simulink library "halin"  (R2021b)
settings: Solver=VariableStepAuto  StartTime=0.0  StopTime=10.0  RelTol=1e-3
undefined symbols (not defined in the file): TRUE
libraries: FVT_lib x100, hcu_lib x41
(part 4 of 10)

== system halin/HAL_IN/CAN1/EBC5 ==
  DT_CAN1_SG_EBC5 : Inport
  BrkTempeWarn : Subsystem
  FndBrkUse : Subsystem
  HaltBrkMode : Subsystem
  HillHolderMode : Subsystem
  ParkBrkActuFAct : Subsystem
  XBRAcltnLimit : Subsystem
  XBRActtrlMode : Subsystem
  XBRSysSta : Subsystem
  bus_selector : BusSelector  OutputSignals=CAN1_BrkTempeWarn
  bus_selector1 : BusSelector  OutputSignals=CAN1_FndBrkUse
  bus_selector2 : BusSelector  OutputSignals=CAN1_HaltBrkMode
  bus_selector3 : BusSelector  OutputSignals=CAN1_HillHolderMode
  bus_selector4 : BusSelector  OutputSignals=CAN1_ParkBrkActuFAct
  bus_selector5 : BusSelector  OutputSignals=CAN1_XBRAcltnLimit
  bus_selector6 : BusSelector  OutputSignals=CAN1_XBRActtrlMode
  bus_selector7 : BusSelector  OutputSignals=CAN1_XBRSysSta
  VHAL_BrkTempeWarn_enum : Outport
  VHAL_FndBrkUse_enum : Outport  Port=2
  VHAL_HaltBrkMode_enum : Outport  Port=3
  VHAL_HillHolderMode_enum : Outport  Port=4
  VHAL_ParkBrkActuFAct_enum : Outport  Port=5
  VHAL_XBRAcltnLimit_mps2 : Outport  Port=6
  VHAL_XBRActtrlMode_enum : Outport  Port=7
  VHAL_XBRSysSta_enum : Outport  Port=8
  wires:
  DT_CAN1_SG_EBC5/1 -> [DT_CAN1_SG_EBC5]
  [DT_CAN1_SG_EBC5] -> bus_selector/1
  bus_selector/1 -> BrkTempeWarn/1(BrkTempeWarn)  "<CAN1_BrkTempeWarn>"
  BrkTempeWarn/1(VHAL_BrkTempeWarn_enum) -> VHAL_BrkTempeWarn_enum/1
  [DT_CAN1_SG_EBC5] -> bus_selector1/1
  bus_selector1/1 -> FndBrkUse/1(FndBrkUse)  "<CAN1_FndBrkUse>"
  FndBrkUse/1(VHAL_FndBrkUse_enum) -> VHAL_FndBrkUse_enum/1
  [DT_CAN1_SG_EBC5] -> bus_selector2/1
  bus_selector2/1 -> HaltBrkMode/1(HaltBrkMode)  "<CAN1_HaltBrkMode>"
  HaltBrkMode/1(VHAL_HaltBrkMode_enum) -> VHAL_HaltBrkMode_enum/1
  [DT_CAN1_SG_EBC5] -> bus_selector3/1
  bus_selector3/1 -> HillHolderMode/1(HillHolderMode)  "<CAN1_HillHolderMode>"
  HillHolderMode/1(VHAL_HillHolderMode_enum) -> VHAL_HillHolderMode_enum/1
  [DT_CAN1_SG_EBC5] -> bus_selector4/1
  bus_selector4/1 -> ParkBrkActuFAct/1(ParkBrkActuFAct)  "<CAN1_ParkBrkActuFAct>"
  ParkBrkActuFAct/1(VHAL_ParkBrkActuFAct_enum) -> VHAL_ParkBrkActuFAct_enum/1
  [DT_CAN1_SG_EBC5] -> bus_selector5/1
  bus_selector5/1 -> XBRAcltnLimit/1(XBRAcltnLimit)  "<CAN1_XBRAcltnLimit>"
  XBRAcltnLimit/1(VHAL_XBRAcltnLimit_mps2) -> VHAL_XBRAcltnLimit_mps2/1
  [DT_CAN1_SG_EBC5] -> bus_selector6/1
  bus_selector6/1 -> XBRActtrlMode/1(XBRActtrlMode)  "<CAN1_XBRActtrlMode>"
  XBRActtrlMode/1(VHAL_XBRActtrlMode_enum) -> VHAL_XBRActtrlMode_enum/1
  [DT_CAN1_SG_EBC5] -> bus_selector7/1
  bus_selector7/1 -> XBRSysSta/1(XBRSysSta)  "<CAN1_XBRSysSta>"
  XBRSysSta/1(VHAL_XBRSysSta_enum) -> VHAL_XBRSysSta_enum/1

== system halin/HAL_IN/CAN1/EHPS_Status_1 ==
  DT_CAN1_SG_EHPS_Status_1 : Inport
  EHPSEnSta : Subsystem
  bus_selector : BusSelector  OutputSignals=CAN1_EHPSEnSta
  VHAL_EHPSEnSta_enum : Outport
  wires:
  DT_CAN1_SG_EHPS_Status_1/1 -> [DT_CAN1_SG_EHPS_Status_1]
  [DT_CAN1_SG_EHPS_Status_1] -> bus_selector/1
  bus_selector/1 -> EHPSEnSta/1(EHPSEnSta)  "<CAN1_EHPSEnSta>"
  EHPSEnSta/1(VHAL_EHPSEnSta_enum) -> VHAL_EHPSEnSta_enum/1

== system halin/HAL_IN/CAN1/EMC1_EM1 ==
  DT_CAN1_SG_EMC1_EM1 : Inport
  EM1CS : Subsystem
  EM1Cnt : Subsystem
  EM1OvrCtrlMBrk : Subsystem
  EM1OvrCtrlMDriv : Subsystem
  EM1OvrCtrlMPriBrk : Subsystem
  EM1OvrCtrlMPriDriv : Subsystem
  EM1ReqTorqHRlsBrk : Subsystem
  EM1ReqTorqHRlsDri : Subsystem
  EM1ReqTorqLimBrk : Subsystem
  EM1ReqTorqLimDriv : Subsystem
  bus_selector : BusSelector  OutputSignals=CAN1_EM1CS
  bus_selector1 : BusSelector  OutputSignals=CAN1_EM1Cnt
  bus_selector2 : BusSelector  OutputSignals=CAN1_EM1OvrCtrlMBrk
  bus_selector3 : BusSelector  OutputSignals=CAN1_EM1OvrCtrlMDriv
  bus_selector4 : BusSelector  OutputSignals=CAN1_EM1OvrCtrlMPriBrk
  bus_selector5 : BusSelector  OutputSignals=CAN1_EM1OvrCtrlMPriDriv
  bus_selector6 : BusSelector  OutputSignals=CAN1_EM1ReqTorqHRlsBrk
  bus_selector7 : BusSelector  OutputSignals=CAN1_EM1ReqTorqHRlsDri
  bus_selector8 : BusSelector  OutputSignals=CAN1_EM1ReqTorqLimBrk
  bus_selector9 : BusSelector  OutputSignals=CAN1_EM1ReqTorqLimDriv
  VHAL_EM1CS_enum : Outport
  VHAL_EM1Cnt_enum : Outport  Port=2
  VHAL_EM1OvrCtrlMBrk_enum : Outport  Port=3
  VHAL_EM1OvrCtrlMDriv_enum : Outport  Port=4
  VHAL_EM1OvrCtrlMPriBrk_enum : Outport  Port=5
  VHAL_EM1OvrCtrlMPriDriv_enum : Outport  Port=6
  VHAL_EM1ReqTorqHRlsBrk_pct : Outport  Port=7
  VHAL_EM1ReqTorqHRlsDri_pct : Outport  Port=8
  VHAL_EM1ReqTorqLimBrk_pct : Outport  Port=9
  VHAL_EM1ReqTorqLimDriv_pct : Outport  Port=10
  wires:
  DT_CAN1_SG_EMC1_EM1/1 -> [DT_CAN1_SG_EMC1_EM1]
  [DT_CAN1_SG_EMC1_EM1] -> bus_selector/1
  bus_selector/1 -> EM1CS/1(EM1CS)  "<CAN1_EM1CS>"
  EM1CS/1(VHAL_EM1CS_enum) -> VHAL_EM1CS_enum/1
  [DT_CAN1_SG_EMC1_EM1] -> bus_selector1/1
  bus_selector1/1 -> EM1Cnt/1(EM1Cnt)  "<CAN1_EM1Cnt>"
  EM1Cnt/1(VHAL_EM1Cnt_enum) -> VHAL_EM1Cnt_enum/1
  [DT_CAN1_SG_EMC1_EM1] -> bus_selector2/1
  bus_selector2/1 -> EM1OvrCtrlMBrk/1(EM1OvrCtrlMBrk)  "<CAN1_EM1OvrCtrlMBrk>"
  EM1OvrCtrlMBrk/1(VHAL_EM1OvrCtrlMBrk_enum) -> VHAL_EM1OvrCtrlMBrk_enum/1
  [DT_CAN1_SG_EMC1_EM1] -> bus_selector3/1
  bus_selector3/1 -> EM1OvrCtrlMDriv/1(EM1OvrCtrlMDriv)  "<CAN1_EM1OvrCtrlMDriv>"
  EM1OvrCtrlMDriv/1(VHAL_EM1OvrCtrlMDriv_enum) -> VHAL_EM1OvrCtrlMDriv_enum/1
  [DT_CAN1_SG_EMC1_EM1] -> bus_selector4/1
  bus_selector4/1 -> EM1OvrCtrlMPriBrk/1(EM1OvrCtrlMPriBrk)  "<CAN1_EM1OvrCtrlMPriBrk>"
  EM1OvrCtrlMPriBrk/1(VHAL_EM1OvrCtrlMPriBrk_enum) -> VHAL_EM1OvrCtrlMPriBrk_enum/1
  [DT_CAN1_SG_EMC1_EM1] -> bus_selector5/1
  bus_selector5/1 -> EM1OvrCtrlMPriDriv/1(EM1OvrCtrlMPriDriv)  "<CAN1_EM1OvrCtrlMPriDriv>"
  EM1OvrCtrlMPriDriv/1(VHAL_EM1OvrCtrlMPriDriv_enum) -> VHAL_EM1OvrCtrlMPriDriv_enum/1
  [DT_CAN1_SG_EMC1_EM1] -> bus_selector6/1
  bus_selector6/1 -> EM1ReqTorqHRlsBrk/1(EM1ReqTorqHRlsBrk)  "<CAN1_EM1ReqTorqHRlsBrk>"
  EM1ReqTorqHRlsBrk/1(VHAL_EM1ReqTorqHRlsBrk_pct) -> VHAL_EM1ReqTorqHRlsBrk_pct/1
  [DT_CAN1_SG_EMC1_EM1] -> bus_selector7/1
  bus_selector7/1 -> EM1ReqTorqHRlsDri/1(EM1ReqTorqHRlsDri)  "<CAN1_EM1ReqTorqHRlsDri>"
  EM1ReqTorqHRlsDri/1(VHAL_EM1ReqTorqHRlsDri_pct) -> VHAL_EM1ReqTorqHRlsDri_pct/1
  [DT_CAN1_SG_EMC1_EM1] -> bus_selector8/1
  bus_selector8/1 -> EM1ReqTorqLimBrk/1(EM1ReqTorqLimBrk)  "<CAN1_EM1ReqTorqLimBrk>"
  EM1ReqTorqLimBrk/1(VHAL_EM1ReqTorqLimBrk_pct) -> VHAL_EM1ReqTorqLimBrk_pct/1
  [DT_CAN1_SG_EMC1_EM1] -> bus_selector9/1
  bus_selector9/1 -> EM1ReqTorqLimDriv/1(EM1ReqTorqLimDriv)  "<CAN1_EM1ReqTorqLimDriv>"
  EM1ReqTorqLimDriv/1(VHAL_EM1ReqTorqLimDriv_pct) -> VHAL_EM1ReqTorqLimDriv_pct/1

== system halin/HAL_IN/CAN1/EPB1 ==
  DT_CAN1_SG_EPB1 : Inport
  EPBParkingBrakeSta : Subsystem
  bus_selector : BusSelector  OutputSignals=CAN1_EPB_ParkingBrake_Sta
  VHAL_EPBParkingBrakeSta_enum : Outport
  wires:
  DT_CAN1_SG_EPB1/1 -> [DT_CAN1_SG_EPB1]
  [DT_CAN1_SG_EPB1] -> bus_selector/1
  bus_selector/1 -> EPBParkingBrakeSta/1(EPB_ParkingBrake_Sta)  "<CAN1_EPB_ParkingBrake_Sta>"
  EPBParkingBrakeSta/1(VHAL_EPBParkingBrakeSta_enum) -> VHAL_EPBParkingBrakeSta_enum/1

== system halin/HAL_IN/CAN1/PDU_Status_1 ==
  DT_CAN1_SG_PDU_Status_1 : Inport
  PDUDCDCRlySta : Subsystem
  PDUEACRlySta : Subsystem
  PDUEHPSRlySta : Subsystem
  PDUSelfChkSta : Subsystem
  bus_selector : BusSelector  OutputSignals=CAN1_PDUDCDCRlySta
  bus_selector1 : BusSelector  OutputSignals=CAN1_PDUEACRlySta
  bus_selector2 : BusSelector  OutputSignals=CAN1_PDUEHPSRlySta
  bus_selector3 : BusSelector  OutputSignals=CAN1_PDUSelfChkSta
  VHAL_PDUDCDCRlySta_enum : Outport
  VHAL_PDUEACRlySta_enum : Outport  Port=2
  VHAL_PDUEHPSRlySta_enum : Outport  Port=3
  VHAL_PDUSelfChkSta_enum : Outport  Port=4
  wires:
  DT_CAN1_SG_PDU_Status_1/1 -> [DT_CAN1_SG_PDU_Status_1]
  [DT_CAN1_SG_PDU_Status_1] -> bus_selector/1
  bus_selector/1 -> PDUDCDCRlySta/1(PDUDCDCRlySta)  "<CAN1_PDUDCDCRlySta>"
  PDUDCDCRlySta/1(VHAL_PDUDCDCRlySta_enum) -> VHAL_PDUDCDCRlySta_enum/1
  [DT_CAN1_SG_PDU_Status_1] -> bus_selector1/1
  bus_selector1/1 -> PDUEACRlySta/1(PDUEACRlySta)  "<CAN1_PDUEACRlySta>"
  PDUEACRlySta/1(VHAL_PDUEACRlySta_enum) -> VHAL_PDUEACRlySta_enum/1
  [DT_CAN1_SG_PDU_Status_1] -> bus_selector2/1
  bus_selector2/1 -> PDUEHPSRlySta/1(PDUEHPSRlySta)  "<CAN1_PDUEHPSRlySta>"
  PDUEHPSRlySta/1(VHAL_PDUEHPSRlySta_enum) -> VHAL_PDUEHPSRlySta_enum/1
  [DT_CAN1_SG_PDU_Status_1] -> bus_selector3/1
  bus_selector3/1 -> PDUSelfChkSta/1(PDUSelfChkSta)  "<CAN1_PDUSelfChkSta>"
  PDUSelfChkSta/1(VHAL_PDUSelfChkSta_enum) -> VHAL_PDUSelfChkSta_enum/1

== system halin/HAL_IN/CAN1/VHAL_CANMsgInvalidDCDCStatus1_flg ==
  Cast To Boolean13 : DataTypeConversion  OutDataTypeStr=boolean
  Constant : Constant  Value=TRUE
  Latch13 : hcu_lib/Basic_Blocks/Latch
  Switch13 : Switch  Criteria=u2 ~= 0
  Unit Delay : UnitDelay  SampleTime=-1  HasFrameUpgradeWarning=on
  UnitConverter : DataTypeConversion  OutDataTypeStr=boolean
  Out : Outport
  wires:
  Constant/1 -> Switch13/3
  Unit Delay/1 -> Cast To Boolean13/1
  Cast To Boolean13/1 -> Switch13/1, Latch13/1
  Switch13/1 -> UnitConverter/1
  Latch13/1 -> Switch13/2
  UnitConverter/1 -> Unit Delay/1, Out/1  "VHAL_CANMsgInvalidDCDCStatus1_flg"

== system halin/HAL_IN/CAN1/VHAL_CANMsgInvalidDCDCStatus2_flg ==
  Cast To Boolean13 : DataTypeConversion  OutDataTypeStr=boolean
  Constant : Constant  Value=TRUE
  Latch13 : hcu_lib/Basic_Blocks/Latch
  Switch13 : Switch  Criteria=u2 ~= 0
  Unit Delay : UnitDelay  SampleTime=-1  HasFrameUpgradeWarning=on
  UnitConverter : DataTypeConversion  OutDataTypeStr=boolean
  Out : Outport
  wires:
  Constant/1 -> Switch13/3
  Unit Delay/1 -> Cast To Boolean13/1
  Cast To Boolean13/1 -> Switch13/1, Latch13/1
  Switch13/1 -> UnitConverter/1
  Latch13/1 -> Switch13/2
  UnitConverter/1 -> Unit Delay/1, Out/1  "VHAL_CANMsgInvalidDCDCStatus2_flg"

== system halin/HAL_IN/CAN1/VHAL_CANMsgInvalidEACStatus1_flg ==
  Cast To Boolean13 : DataTypeConversion  OutDataTypeStr=boolean
  Constant : Constant  Value=TRUE
  Latch13 : hcu_lib/Basic_Blocks/Latch
  Switch13 : Switch  Criteria=u2 ~= 0
  Unit Delay : UnitDelay  SampleTime=-1  HasFrameUpgradeWarning=on
  UnitConverter : DataTypeConversion  OutDataTypeStr=boolean
  Out : Outport
  wires:
  Constant/1 -> Switch13/3
  Unit Delay/1 -> Cast To Boolean13/1
  Cast To Boolean13/1 -> Switch13/1, Latch13/1
  Switch13/1 -> UnitConverter/1
  Latch13/1 -> Switch13/2
  UnitConverter/1 -> Unit Delay/1, Out/1  "VHAL_CANMsgInvalidEACStatus1_flg"

== system halin/HAL_IN/CAN1/VHAL_CANMsgInvalidEBC1_flg ==
  Cast To Boolean13 : DataTypeConversion  OutDataTypeStr=boolean
  Constant : Constant  Value=TRUE
  Latch13 : hcu_lib/Basic_Blocks/Latch
  Switch13 : Switch  Criteria=u2 ~= 0
  Unit Delay : UnitDelay  SampleTime=-1  HasFrameUpgradeWarning=on
  UnitConverter : DataTypeConversion  OutDataTypeStr=boolean
  Out : Outport
  wires:
  Constant/1 -> Switch13/3
  Unit Delay/1 -> Cast To Boolean13/1
  Cast To Boolean13/1 -> Switch13/1, Latch13/1
  Switch13/1 -> UnitConverter/1
  Latch13/1 -> Switch13/2
  UnitConverter/1 -> Unit Delay/1, Out/1  "VHAL_CANMsgInvalidEBC1_flg"

== system halin/HAL_IN/CAN1/VHAL_CANMsgInvalidEBC2_flg ==
  Cast To Boolean13 : DataTypeConversion  OutDataTypeStr=boolean
  Constant : Constant  Value=TRUE
  Latch13 : hcu_lib/Basic_Blocks/Latch
  Switch13 : Switch  Criteria=u2 ~= 0
  Unit Delay : UnitDelay  SampleTime=-1  HasFrameUpgradeWarning=on
  UnitConverter : DataTypeConversion  OutDataTypeStr=boolean
  Out : Outport
  wires:
  Constant/1 -> Switch13/3
  Unit Delay/1 -> Cast To Boolean13/1
  Cast To Boolean13/1 -> Switch13/1, Latch13/1
  Switch13/1 -> UnitConverter/1
  Latch13/1 -> Switch13/2
  UnitConverter/1 -> Unit Delay/1, Out/1  "VHAL_CANMsgInvalidEBC2_flg"

== system halin/HAL_IN/CAN1/VHAL_CANMsgInvalidEBC5_flg ==
  Cast To Boolean13 : DataTypeConversion  OutDataTypeStr=boolean
  Constant : Constant  Value=TRUE
  Latch13 : hcu_lib/Basic_Blocks/Latch
  Switch13 : Switch  Criteria=u2 ~= 0
  Unit Delay : UnitDelay  SampleTime=-1  HasFrameUpgradeWarning=on
  UnitConverter : DataTypeConversion  OutDataTypeStr=boolean
  Out : Outport
  wires:
  Constant/1 -> Switch13/3
  Unit Delay/1 -> Cast To Boolean13/1
  Cast To Boolean13/1 -> Switch13/1, Latch13/1
  Switch13/1 -> UnitConverter/1
  Latch13/1 -> Switch13/2
  UnitConverter/1 -> Unit Delay/1, Out/1  "VHAL_CANMsgInvalidEBC5_flg"

== system halin/HAL_IN/CAN1/VHAL_CANMsgInvalidEHPSStatus1_flg ==
  Cast To Boolean13 : DataTypeConversion  OutDataTypeStr=boolean
  Constant : Constant  Value=TRUE
  Latch13 : hcu_lib/Basic_Blocks/Latch
  Switch13 : Switch  Criteria=u2 ~= 0
  Unit Delay : UnitDelay  SampleTime=-1  HasFrameUpgradeWarning=on
  UnitConverter : DataTypeConversion  OutDataTypeStr=boolean
  Out : Outport
  wires:
  Constant/1 -> Switch13/3
  Unit Delay/1 -> Cast To Boolean13/1
  Cast To Boolean13/1 -> Switch13/1, Latch13/1
  Switch13/1 -> UnitConverter/1
  Latch13/1 -> Switch13/2
  UnitConverter/1 -> Unit Delay/1, Out/1  "VHAL_CANMsgInvalidEHPSStatus1_flg"

== system halin/HAL_IN/CAN1/VHAL_CANMsgInvalidEMC1EM1_flg ==
  Cast To Boolean13 : DataTypeConversion  OutDataTypeStr=boolean
  Constant : Constant  Value=TRUE
  Latch13 : hcu_lib/Basic_Blocks/Latch
  Switch13 : Switch  Criteria=u2 ~= 0
  Unit Delay : UnitDelay  SampleTime=-1  HasFrameUpgradeWarning=on
  UnitConverter : DataTypeConversion  OutDataTypeStr=boolean
  Out : Outport
  wires:
  Constant/1 -> Switch13/3
  Unit Delay/1 -> Cast To Boolean13/1
  Cast To Boolean13/1 -> Switch13/1, Latch13/1
  Switch13/1 -> UnitConverter/1
  Latch13/1 -> Switch13/2
  UnitConverter/1 -> Unit Delay/1, Out/1  "VHAL_CANMsgInvalidEMC1EM1_flg"

== system halin/HAL_IN/CAN1/VHAL_CANMsgInvalidEPB1_flg ==
  Cast To Boolean13 : DataTypeConversion  OutDataTypeStr=boolean
  Constant : Constant  Value=TRUE
  Latch13 : hcu_lib/Basic_Blocks/Latch
  Switch13 : Switch  Criteria=u2 ~= 0
  Unit Delay : UnitDelay  SampleTime=-1  HasFrameUpgradeWarning=on
  UnitConverter : DataTypeConversion  OutDataTypeStr=boolean
  Out : Outport
  wires:
  Constant/1 -> Switch13/3
  Unit Delay/1 -> Cast To Boolean13/1
  Cast To Boolean13/1 -> Switch13/1, Latch13/1
  Switch13/1 -> UnitConverter/1
  Latch13/1 -> Switch13/2
  UnitConverter/1 -> Unit Delay/1, Out/1  "VHAL_CANMsgInvalidEPB1_flg"

== system halin/HAL_IN/CAN1/VHAL_CANMsgInvalidPDUStatus1_flg ==
  Cast To Boolean13 : DataTypeConversion  OutDataTypeStr=boolean
  Constant : Constant  Value=TRUE
  Latch13 : hcu_lib/Basic_Blocks/Latch
  Switch13 : Switch  Criteria=u2 ~= 0
  Unit Delay : UnitDelay  SampleTime=-1  HasFrameUpgradeWarning=on
  UnitConverter : DataTypeConversion  OutDataTypeStr=boolean
  Out : Outport
  wires:
  Constant/1 -> Switch13/3
  Unit Delay/1 -> Cast To Boolean13/1
  Cast To Boolean13/1 -> Switch13/1, Latch13/1
  Switch13/1 -> UnitConverter/1
  Latch13/1 -> Switch13/2
  UnitConverter/1 -> Unit Delay/1, Out/1  "VHAL_CANMsgInvalidPDUStatus1_flg"

== system halin/HAL_IN/CAN2/IVI1 ==
  DT_CAN2_SG_IVI1 : Inport
  AmbLighLowBatAlertSW : Subsystem
  AmbLighSafetyAlertSW : Subsystem
  AmbLightColorSet : Subsystem
  AmbLightDimInDarkSW : Subsystem
  AmbLightSW : Subsystem
  AmbLightWlcmLightSW : Subsystem
  FCPFrEvtBtnACMaxReq : Subsystem
  FCPFrEvtBtnACReq : Subsystem
  FCPFrEvtBtnAutoReq : Subsystem
  FCPFrEvtBtnSyncReq : Subsystem
  IVITimeCheck : Subsystem
  IVITimeDay : Subsystem
  IVITimeHour : Subsystem
  IVITimeMinute : Subsystem
  IVITimeMonth : Subsystem
  IVITimeSecond : Subsystem
  IVITimeYear : Subsystem
  LINKtoDrive : Subsystem
  OpenDrOpenWdoSW : Subsystem
  PWCONTINUEUSE : Subsystem
  SmartEcoModeSW : Subsystem
  bus_selector : BusSelector  OutputSignals=CAN2_AmbLigh_LowBatAlert_SW
  bus_selector1 : BusSelector  OutputSignals=CAN2_AmbLigh_SafetyAlert_SW
  bus_selector10 : BusSelector  OutputSignals=CAN2_IVI_Time_Check
  bus_selector11 : BusSelector  OutputSignals=CAN2_IVI_Time_Day
  bus_selector12 : BusSelector  OutputSignals=CAN2_IVI_Time_Hour
  bus_selector13 : BusSelector  OutputSignals=CAN2_IVI_Time_Minute
  bus_selector14 : BusSelector  OutputSignals=CAN2_IVI_Time_Month
  bus_selector15 : BusSelector  OutputSignals=CAN2_IVI_Time_Second
  bus_selector16 : BusSelector  OutputSignals=CAN2_IVI_Time_Year
  bus_selector17 : BusSelector  OutputSignals=CAN2_LINKtoDrive
  bus_selector18 : BusSelector  OutputSignals=CAN2_OpenDrOpenWdo_SW
  bus_selector19 : BusSelector  OutputSignals=CAN2_PW_CONTINUE_USE
  bus_selector2 : BusSelector  OutputSignals=CAN2_AmbLightColorSet
  bus_selector20 : BusSelector  OutputSignals=CAN2_SmartEco_Mode_SW
  bus_selector3 : BusSelector  OutputSignals=CAN2_AmbLight_DimInDark_SW
  bus_selector4 : BusSelector  OutputSignals=CAN2_AmbLight_SW
  bus_selector5 : BusSelector  OutputSignals=CAN2_AmbLight_WlcmLight_SW
  bus_selector6 : BusSelector  OutputSignals=CAN2_FCP_FrEvt_BtnACMaxReq
  bus_selector7 : BusSelector  OutputSignals=CAN2_FCP_FrEvt_BtnACReq
  bus_selector8 : BusSelector  OutputSignals=CAN2_FCP_FrEvt_BtnAutoReq
  bus_selector9 : BusSelector  OutputSignals=CAN2_FCP_FrEvt_BtnSyncReq
  VHAL_AmbLighLowBatAlertSW_flg : Outport
  VHAL_AmbLighSafetyAlertSW_flg : Outport  Port=2
  VHAL_AmbLightColorSet_enum : Outport  Port=3
  VHAL_AmbLightDimInDarkSW_flg : Outport  Port=4
  VHAL_AmbLightSW_flg : Outport  Port=5
  VHAL_AmbLightWlcmLightSW_flg : Outport  Port=6
  VHAL_FCPFrEvtBtnACMaxReq_flg : Outport  Port=7
  VHAL_FCPFrEvtBtnACReq_flg : Outport  Port=8
  VHAL_FCPFrEvtBtnAutoReq_flg : Outport  Port=9
  VHAL_FCPFrEvtBtnSyncReq_flg : Outport  Port=10
  VHAL_IVITimeCheck_enum : Outport  Port=11
  VHAL_IVITimeDay_DAY : Outport  Port=12
  VHAL_IVITimeHour_hr : Outport  Port=13
  VHAL_IVITimeMinute_min : Outport  Port=14
  VHAL_IVITimeMonth_MONTH : Outport  Port=15
  VHAL_IVITimeSecond_s : Outport  Port=16
  VHAL_IVITimeYear_YEAR : Outport  Port=17
  VHAL_LINKtoDrive_flg : Outport  Port=18
  VHAL_OpenDrOpenWdoSW_flg : Outport  Port=19
  VHAL_PWCONTINUEUSE_flg : Outport  Port=20
  VHAL_SmartEcoModeSW_flg : Outport  Port=21
  wires:
  DT_CAN2_SG_IVI1/1 -> [DT_CAN2_SG_IVI1]
  [DT_CAN2_SG_IVI1] -> bus_selector/1
  bus_selector/1 -> AmbLighLowBatAlertSW/1(AmbLigh_LowBatAlert_SW)  "<CAN2_AmbLigh_LowBatAlert_SW>"
  AmbLighLowBatAlertSW/1(VHAL_AmbLighLowBatAlertSW_flg) -> VHAL_AmbLighLowBatAlertSW_flg/1
  [DT_CAN2_SG_IVI1] -> bus_selector1/1
  bus_selector1/1 -> AmbLighSafetyAlertSW/1(AmbLigh_SafetyAlert_SW)  "<CAN2_AmbLigh_SafetyAlert_SW>"
  AmbLighSafetyAlertSW/1(VHAL_AmbLighSafetyAlertSW_flg) -> VHAL_AmbLighSafetyAlertSW_flg/1
  [DT_CAN2_SG_IVI1] -> bus_selector2/1
  bus_selector2/1 -> AmbLightColorSet/1(AmbLightColorSet)  "<CAN2_AmbLightColorSet>"
  AmbLightColorSet/1(VHAL_AmbLightColorSet_enum) -> VHAL_AmbLightColorSet_enum/1
  [DT_CAN2_SG_IVI1] -> bus_selector3/1
  bus_selector3/1 -> AmbLightDimInDarkSW/1(AmbLight_DimInDark_SW)  "<CAN2_AmbLight_DimInDark_SW>"
  AmbLightDimInDarkSW/1(VHAL_AmbLightDimInDarkSW_flg) -> VHAL_AmbLightDimInDarkSW_flg/1
  [DT_CAN2_SG_IVI1] -> bus_selector4/1
  bus_selector4/1 -> AmbLightSW/1(AmbLight_SW)  "<CAN2_AmbLight_SW>"
  AmbLightSW/1(VHAL_AmbLightSW_flg) -> VHAL_AmbLightSW_flg/1
  [DT_CAN2_SG_IVI1] -> bus_selector5/1
  bus_selector5/1 -> AmbLightWlcmLightSW/1(AmbLight_WlcmLight_SW)  "<CAN2_AmbLight_WlcmLight_SW>"
  AmbLightWlcmLightSW/1(VHAL_AmbLightWlcmLightSW_flg) -> VHAL_AmbLightWlcmLightSW_flg/1
  [DT_CAN2_SG_IVI1] -> bus_selector6/1
  bus_selector6/1 -> FCPFrEvtBtnACMaxReq/1(FCP_FrEvt_BtnACMaxReq)  "<CAN2_FCP_FrEvt_BtnACMaxReq>"
  FCPFrEvtBtnACMaxReq/1(VHAL_FCPFrEvtBtnACMaxReq_flg) -> VHAL_FCPFrEvtBtnACMaxReq_flg/1
  [DT_CAN2_SG_IVI1] -> bus_selector7/1
  bus_selector7/1 -> FCPFrEvtBtnACReq/1(FCP_FrEvt_BtnACReq)  "<CAN2_FCP_FrEvt_BtnACReq>"
  FCPFrEvtBtnACReq/1(VHAL_FCPFrEvtBtnACReq_flg) -> VHAL_FCPFrEvtBtnACReq_flg/1
  [DT_CAN2_SG_IVI1] -> bus_selector8/1
  bus_selector8/1 -> FCPFrEvtBtnAutoReq/1(FCP_FrEvt_BtnAutoReq)  "<CAN2_FCP_FrEvt_BtnAutoReq>"
  FCPFrEvtBtnAutoReq/1(VHAL_FCPFrEvtBtnAutoReq_flg) -> VHAL_FCPFrEvtBtnAutoReq_flg/1
  [DT_CAN2_SG_IVI1] -> bus_selector9/1
  bus_selector9/1 -> FCPFrEvtBtnSyncReq/1(FCP_FrEvt_BtnSyncReq)  "<CAN2_FCP_FrEvt_BtnSyncReq>"
  FCPFrEvtBtnSyncReq/1(VHAL_FCPFrEvtBtnSyncReq_flg) -> VHAL_FCPFrEvtBtnSyncReq_flg/1
  [DT_CAN2_SG_IVI1] -> bus_selector10/1
  bus_selector10/1 -> IVITimeCheck/1(IVI_Time_Check)  "<CAN2_IVI_Time_Check>"
  IVITimeCheck/1(VHAL_IVITimeCheck_enum) -> VHAL_IVITimeCheck_enum/1
  [DT_CAN2_SG_IVI1] -> bus_selector11/1
  bus_selector11/1 -> IVITimeDay/1(IVI_Time_Day)  "<CAN2_IVI_Time_Day>"
  IVITimeDay/1(VHAL_IVITimeDay_DAY) -> VHAL_IVITimeDay_DAY/1
  [DT_CAN2_SG_IVI1] -> bus_selector12/1
  bus_selector12/1 -> IVITimeHour/1(IVI_Time_Hour)  "<CAN2_IVI_Time_Hour>"
  IVITimeHour/1(VHAL_IVITimeHour_hr) -> VHAL_IVITimeHour_hr/1
  [DT_CAN2_SG_IVI1] -> bus_selector13/1
  bus_selector13/1 -> IVITimeMinute/1(IVI_Time_Minute)  "<CAN2_IVI_Time_Minute>"
  IVITimeMinute/1(VHAL_IVITimeMinute_min) -> VHAL_IVITimeMinute_min/1
  [DT_CAN2_SG_IVI1] -> bus_selector14/1
  bus_selector14/1 -> IVITimeMonth/1(IVI_Time_Month)  "<CAN2_IVI_Time_Month>"
  IVITimeMonth/1(VHAL_IVITimeMonth_MONTH) -> VHAL_IVITimeMonth_MONTH/1
  [DT_CAN2_SG_IVI1] -> bus_selector15/1
  bus_selector15/1 -> IVITimeSecond/1(IVI_Time_Second)  "<CAN2_IVI_Time_Second>"
  IVITimeSecond/1(VHAL_IVITimeSecond_s) -> VHAL_IVITimeSecond_s/1
  [DT_CAN2_SG_IVI1] -> bus_selector16/1
  bus_selector16/1 -> IVITimeYear/1(IVI_Time_Year)  "<CAN2_IVI_Time_Year>"
  IVITimeYear/1(VHAL_IVITimeYear_YEAR) -> VHAL_IVITimeYear_YEAR/1
  [DT_CAN2_SG_IVI1] -> bus_selector17/1
  bus_selector17/1 -> LINKtoDrive/1(LINKtoDrive)  "<CAN2_LINKtoDrive>"
  LINKtoDrive/1(VHAL_LINKtoDrive_flg) -> VHAL_LINKtoDrive_flg/1
  [DT_CAN2_SG_IVI1] -> bus_selector18/1
  bus_selector18/1 -> OpenDrOpenWdoSW/1(OpenDrOpenWdo_SW)  "<CAN2_OpenDrOpenWdo_SW>"
  OpenDrOpenWdoSW/1(VHAL_OpenDrOpenWdoSW_flg) -> VHAL_OpenDrOpenWdoSW_flg/1
  [DT_CAN2_SG_IVI1] -> bus_selector19/1
  bus_selector19/1 -> PWCONTINUEUSE/1(PW_CONTINUE_USE)  "<CAN2_PW_CONTINUE_USE>"
  PWCONTINUEUSE/1(VHAL_PWCONTINUEUSE_flg) -> VHAL_PWCONTINUEUSE_flg/1
  [DT_CAN2_SG_IVI1] -> bus_selector20/1
  bus_selector20/1 -> SmartEcoModeSW/1(SmartEco_Mode_SW)  "<CAN2_SmartEco_Mode_SW>"
  SmartEcoModeSW/1(VHAL_SmartEcoModeSW_flg) -> VHAL_SmartEcoModeSW_flg/1

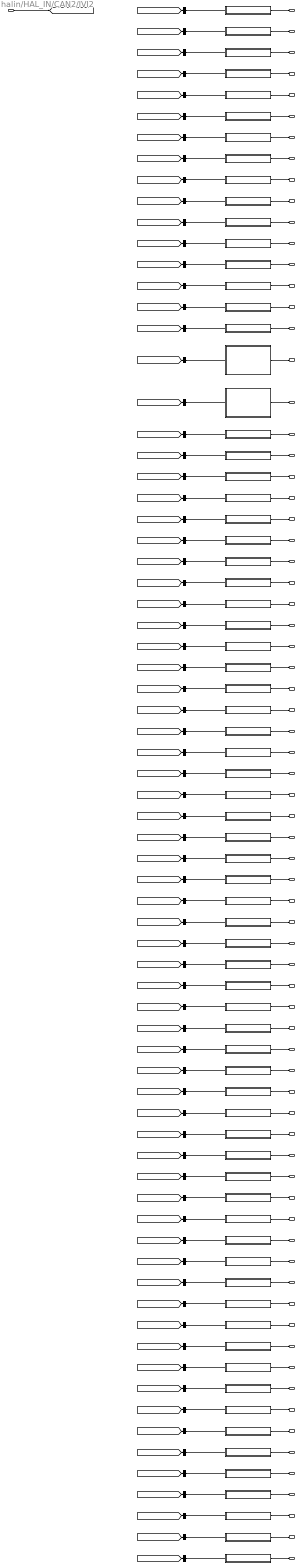
== system halin/HAL_IN/CAN2/IVI2 ==
  DT_CAN2_SG_IVI2 : Inport
  ACChgCurSet : Subsystem
  AVMErrSTA : Subsystem
  AVMOFFRecButt : Subsystem
  AVMParkingmode : Subsystem
  AVMparkingcancel : Subsystem
  AVMparkingexcute : Subsystem
  CAASSw : Subsystem
  CDLLockButt : Subsystem
  CDLUnlockButt : Subsystem
  DSEATantiset : Subsystem
  DSEATentryfunset : Subsystem
  DSEATventreq : Subsystem
  Distanceunit : Subsystem
  ESCSWCmd : Subsystem
  FSOffSw : Subsystem
  FollowMeSW : Subsystem
  GPSLAT : Subsystem
  GPSLONG : Subsystem
  HeadLampSW : Subsystem
  HoodLatchSW : Subsystem
  IVINightModeSta : Subsystem
  IVIPTGModeSW : Subsystem
  IVIPTGStaSW : Subsystem
  IVIPTGUSStaSW : Subsystem
  IVIPWModeReq : Subsystem
  IVIPwrLockSW : Subsystem
  IVIPwroffreq : Subsystem
  IVIRRDefReq : Subsystem
  IVIReqV2L : Subsystem
  IVIScreen : Subsystem
  IVIStartChgreq : Subsystem
  IVIStatus : Subsystem
  IVIStopChgreq : Subsystem
  IVITriggerreq : Subsystem
  IVIUnlockChgreq : Subsystem
  IVIWIMAINSW : Subsystem
  LDrvControlCommand : Subsystem
  LPasControlCommand : Subsystem
  LRLDControlCommand : Subsystem
  LRRDControlCommand : Subsystem
  LightShowStartReq : Subsystem
  LightShowStopReq : Subsystem
  MFRDNBrightReq : Subsystem
  OFFACMODE : Subsystem
  PSEATventreq : Subsystem
  PerdV2L : Subsystem
  RFogLampSW : Subsystem
  RollModeSWCmd : Subsystem
  RoomLampMode : Subsystem
  SOCADJBUTT : Subsystem
  SOCLimitSet : Subsystem
  SOCV2LLimit : Subsystem
  SchedChgStart : Subsystem
  SchedChgStop : Subsystem
  SchedChgbutt : Subsystem
  SchedChglimit : Subsystem
  SchedChgwake : Subsystem
  SenstivityPosition : Subsystem
  SetUnlockSingle : Subsystem
  TCSSWCmd : Subsystem
  TPMSCaliButt : Subsystem
  TPMSResButt : Subsystem
  TurnSwTimeSet : Subsystem
  WalkawayLockSW : Subsystem
  WlcmLightMode : Subsystem
  bus_selector : BusSelector  OutputSignals=CAN2_AC_Chg_Cur_Set
  bus_selector1 : BusSelector  OutputSignals=CAN2_AVM_Err_STA
  bus_selector10 : BusSelector  OutputSignals=CAN2_DSEAT_entryfun_set
  bus_selector11 : BusSelector  OutputSignals=CAN2_DSEAT_vent_req
  bus_selector12 : BusSelector  OutputSignals=CAN2_Distance_unit
  bus_selector13 : BusSelector  OutputSignals=CAN2_ESC_SW_Cmd
  bus_selector14 : BusSelector  OutputSignals=CAN2_FS_Off_Sw
  bus_selector15 : BusSelector  OutputSignals=CAN2_FollowMeSW
  bus_selector16 : BusSelector  OutputSignals=CAN2_GPS_LAT
  bus_selector17 : BusSelector  OutputSignals=CAN2_GPS_LONG
  bus_selector18 : BusSelector  OutputSignals=CAN2_HeadLampSW
  bus_selector19 : BusSelector  OutputSignals=CAN2_Hood_Latch_SW
  bus_selector2 : BusSelector  OutputSignals=CAN2_AVM_OFF_Rec_Butt
  bus_selector20 : BusSelector  OutputSignals=CAN2_IVI_Night_Mode_Sta
  bus_selector21 : BusSelector  OutputSignals=CAN2_IVI_PTG_Mode_SW
  bus_selector22 : BusSelector  OutputSignals=CAN2_IVI_PTG_Sta_SW
  bus_selector23 : BusSelector  OutputSignals=CAN2_IVI_PTG_USSta_SW
  bus_selector24 : BusSelector  OutputSignals=CAN2_IVI_PW_Mode_Req
  bus_selector25 : BusSelector  OutputSignals=CAN2_IVI_PwrLockSW
  bus_selector26 : BusSelector  OutputSignals=CAN2_IVI_Pwroff_req
  bus_selector27 : BusSelector  OutputSignals=CAN2_IVI_RR_Def_Req
  bus_selector28 : BusSelector  OutputSignals=CAN2_IVI_Req_V2L
  bus_selector29 : BusSelector  OutputSignals=CAN2_IVI_Screen
  bus_selector3 : BusSelector  OutputSignals=CAN2_AVM_Parking_mode
  bus_selector30 : BusSelector  OutputSignals=CAN2_IVI_Start_Chg_req
  bus_selector31 : BusSelector  OutputSignals=CAN2_IVI_Status
  bus_selector32 : BusSelector  OutputSignals=CAN2_IVI_Stop_Chg_req
  bus_selector33 : BusSelector  OutputSignals=CAN2_IVI_Trigger_req
  bus_selector34 : BusSelector  OutputSignals=CAN2_IVI_Unlock_Chg_req
  bus_selector35 : BusSelector  OutputSignals=CAN2_IVI_WI_MAIN_SW
  bus_selector36 : BusSelector  OutputSignals=CAN2_L_Drv_ControlCommand
  bus_selector37 : BusSelector  OutputSignals=CAN2_L_Pas_ControlCommand
  bus_selector38 : BusSelector  OutputSignals=CAN2_L_RLD_ControlCommand
  bus_selector39 : BusSelector  OutputSignals=CAN2_L_RRD_ControlCommand
  bus_selector4 : BusSelector  OutputSignals=CAN2_AVM_parking_cancel
  bus_selector40 : BusSelector  OutputSignals=CAN2_Light_ShowStart_Req
  bus_selector41 : BusSelector  OutputSignals=CAN2_Light_ShowStop_Req
  bus_selector42 : BusSelector  OutputSignals=CAN2_MFRD_N_Bright_Req
  bus_selector43 : BusSelector  OutputSignals=CAN2_OFF_AC_MODE
  bus_selector44 : BusSelector  OutputSignals=CAN2_PSEAT_vent_req
  bus_selector45 : BusSelector  OutputSignals=CAN2_Perd_V2L
  bus_selector46 : BusSelector  OutputSignals=CAN2_RFogLampSW
  bus_selector47 : BusSelector  OutputSignals=CAN2_Roll_Mode_SW_Cmd
  bus_selector48 : BusSelector  OutputSignals=CAN2_RoomLampMode
  bus_selector49 : BusSelector  OutputSignals=CAN2_SOC_ADJ_BUTT
  bus_selector5 : BusSelector  OutputSignals=CAN2_AVM_parking_excute
  bus_selector50 : BusSelector  OutputSignals=CAN2_SOC_Limit_Set
  bus_selector51 : BusSelector  OutputSignals=CAN2_SOC_V2LLimit
  bus_selector52 : BusSelector  OutputSignals=CAN2_Sched_Chg_Start
  bus_selector53 : BusSelector  OutputSignals=CAN2_Sched_Chg_Stop
  bus_selector54 : BusSelector  OutputSignals=CAN2_Sched_Chg_butt
  bus_selector55 : BusSelector  OutputSignals=CAN2_Sched_Chg_limit
  bus_selector56 : BusSelector  OutputSignals=CAN2_Sched_Chg_wake
  bus_selector57 : BusSelector  OutputSignals=CAN2_SenstivityPosition
  bus_selector58 : BusSelector  OutputSignals=CAN2_SetUnlockSingle
  bus_selector59 : BusSelector  OutputSignals=CAN2_TCS_SW_Cmd
  bus_selector6 : BusSelector  OutputSignals=CAN2_CAAS_Sw
  bus_selector60 : BusSelector  OutputSignals=CAN2_TPMS_Cali_Butt
  bus_selector61 : BusSelector  OutputSignals=CAN2_TPMS_Res_Butt
  bus_selector62 : BusSelector  OutputSignals=CAN2_TurnSwTimeSet
  bus_selector63 : BusSelector  OutputSignals=CAN2_Walkaway_Lock_SW
  bus_selector64 : BusSelector  OutputSignals=CAN2_WlcmLight_Mode
  bus_selector65 : BusSelector  OutputSignals=CAN2_sigAirIntenZon1Req
  bus_selector66 : BusSelector  OutputSignals=CAN2_sigDfrstReq
  bus_selector67 : BusSelector  OutputSignals=CAN2_sigFaceReq
  bus_selector68 : BusSelector  OutputSignals=CAN2_sigFootReq
  bus_selector69 : BusSelector  OutputSignals=CAN2_sigRecircReq
  bus_selector7 : BusSelector  OutputSignals=CAN2_CDL_Lock_Butt
  bus_selector70 : BusSelector  OutputSignals=CAN2_sigSetTempZon1Req
  bus_selector71 : BusSelector  OutputSignals=CAN2_sigSetTempZon2Req
  bus_selector8 : BusSelector  OutputSignals=CAN2_CDL_Unlock_Butt
  bus_selector9 : BusSelector  OutputSignals=CAN2_DSEAT_anti_set
  sigAirIntenZon1Req : Subsystem
  sigDfrstReq : Subsystem
  sigFaceReq : Subsystem
  sigFootReq : Subsystem
  sigRecircReq : Subsystem
  sigSetTempZon1Req : Subsystem
  sigSetTempZon2Req : Subsystem
  VHAL_ACChgCurSet_A : Outport
  VHAL_AVMErrSTA_flg : Outport  Port=2
  VHAL_AVMOFFRecButt_flg : Outport  Port=3
  VHAL_AVMParkingmode_enum : Outport  Port=4
  VHAL_AVMparkingcancel_enum : Outport  Port=5
  VHAL_AVMparkingexcute_enum : Outport  Port=6
  VHAL_CAASSw_enum : Outport  Port=7
  VHAL_CDLLockButt_flg : Outport  Port=8
  VHAL_CDLUnlockButt_flg : Outport  Port=9
  VHAL_DSEATantiset_flg : Outport  Port=10
  VHAL_DSEATentryfunset_flg : Outport  Port=11
  VHAL_DSEATventreq_enum : Outport  Port=12
  VHAL_Distanceunit_flg : Outport  Port=13
  VHAL_ESCSWCmd_enum : Outport  Port=14
  VHAL_FSOffSw_enum : Outport  Port=15
  VHAL_FollowMeSW_flg : Outport  Port=16
  VHAL_GPSLAT_s : Outport  Port=17
  VHAL_GPSLONG_enum : Outport  Port=18
  VHAL_HeadLampSW_enum : Outport  Port=19
  VHAL_HoodLatchSW_enum : Outport  Port=20
  VHAL_IVINightModeSta_flg : Outport  Port=21
  VHAL_IVIPTGModeSW_enum : Outport  Port=22
  VHAL_IVIPTGStaSW_enum : Outport  Port=23
  VHAL_IVIPTGUSStaSW_flg : Outport  Port=24
  VHAL_IVIPWModeReq_enum : Outport  Port=25
  VHAL_IVIPwrLockSW_enum : Outport  Port=26
  VHAL_IVIPwroffreq_flg : Outport  Port=27
  VHAL_IVIRRDefReq_flg : Outport  Port=28
  VHAL_IVIReqV2L_enum : Outport  Port=29
  VHAL_IVIScreen_enum : Outport  Port=30
  VHAL_IVIStartChgreq_flg : Outport  Port=31
  VHAL_IVIStatus_flg : Outport  Port=32
  VHAL_IVIStopChgreq_flg : Outport  Port=33
  VHAL_IVITriggerreq_flg : Outport  Port=34
  VHAL_IVIUnlockChgreq_flg : Outport  Port=35
  VHAL_IVIWIMAINSW_flg : Outport  Port=36
  VHAL_LDrvControlCommand_pct : Outport  Port=37
  VHAL_LPasControlCommand_pct : Outport  Port=38
  VHAL_LRLDControlCommand_pct : Outport  Port=39
  VHAL_LRRDControlCommand_pct : Outport  Port=40
  VHAL_LightShowStartReq_flg : Outport  Port=41
  VHAL_LightShowStopReq_flg : Outport  Port=42
  VHAL_MFRDNBrightReq_pct : Outport  Port=43
  VHAL_OFFACMODE_enum : Outport  Port=44
  VHAL_PSEATventreq_enum : Outport  Port=45
  VHAL_PerdV2L_enum : Outport  Port=46
  VHAL_RFogLampSW_flg : Outport  Port=47
  VHAL_RollModeSWCmd_enum : Outport  Port=48
  VHAL_RoomLampMode_flg : Outport  Port=49
  VHAL_SOCADJBUTT_flg : Outport  Port=50
  VHAL_SOCLimitSet_pct : Outport  Port=51
  VHAL_SOCV2LLimit_pct : Outport  Port=52
  VHAL_SchedChgStart_flg : Outport  Port=53
  VHAL_SchedChgStop_flg : Outport  Port=54
  VHAL_SchedChgbutt_flg : Outport  Port=55
  VHAL_SchedChglimit_pct : Outport  Port=56
  VHAL_SchedChgwake_flg : Outport  Port=57
  VHAL_SenstivityPosition_enum : Outport  Port=58
  VHAL_SetUnlockSingle_flg : Outport  Port=59
  VHAL_TCSSWCmd_enum : Outport  Port=60
  VHAL_TPMSCaliButt_flg : Outport  Port=61
  VHAL_TPMSResButt_flg : Outport  Port=62
  VHAL_TurnSwTimeSet_enum : Outport  Port=63
  VHAL_WalkawayLockSW_flg : Outport  Port=64
  VHAL_WlcmLightMode_enum : Outport  Port=65
  VHAL_sigAirIntenZon1Req_enum : Outport  Port=66
  VHAL_sigDfrstReq_flg : Outport  Port=67
  VHAL_sigFaceReq_flg : Outport  Port=68
  VHAL_sigFootReq_flg : Outport  Port=69
  VHAL_sigRecircReq_flg : Outport  Port=70
  VHAL_sigSetTempZon1Req_C : Outport  Port=71
  VHAL_sigSetTempZon2Req_C : Outport  Port=72
  wires:
  DT_CAN2_SG_IVI2/1 -> [DT_CAN2_SG_IVI2]
  [DT_CAN2_SG_IVI2] -> bus_selector/1
  bus_selector/1 -> ACChgCurSet/1(AC_Chg_Cur_Set)  "<CAN2_AC_Chg_Cur_Set>"
  ACChgCurSet/1(VHAL_ACChgCurSet_A) -> VHAL_ACChgCurSet_A/1
  [DT_CAN2_SG_IVI2] -> bus_selector1/1
  bus_selector1/1 -> AVMErrSTA/1(AVM_Err_STA)  "<CAN2_AVM_Err_STA>"
  AVMErrSTA/1(VHAL_AVMErrSTA_flg) -> VHAL_AVMErrSTA_flg/1
  [DT_CAN2_SG_IVI2] -> bus_selector2/1
  bus_selector2/1 -> AVMOFFRecButt/1(AVM_OFF_Rec_Butt)  "<CAN2_AVM_OFF_Rec_Butt>"
  AVMOFFRecButt/1(VHAL_AVMOFFRecButt_flg) -> VHAL_AVMOFFRecButt_flg/1
  [DT_CAN2_SG_IVI2] -> bus_selector3/1
  bus_selector3/1 -> AVMParkingmode/1(AVM_Parking_mode)  "<CAN2_AVM_Parking_mode>"
  AVMParkingmode/1(VHAL_AVMParkingmode_enum) -> VHAL_AVMParkingmode_enum/1
  [DT_CAN2_SG_IVI2] -> bus_selector4/1
  bus_selector4/1 -> AVMparkingcancel/1(AVM_parking_cancel)  "<CAN2_AVM_parking_cancel>"
  AVMparkingcancel/1(VHAL_AVMparkingcancel_enum) -> VHAL_AVMparkingcancel_enum/1
  [DT_CAN2_SG_IVI2] -> bus_selector5/1
  bus_selector5/1 -> AVMparkingexcute/1(AVM_parking_excute)  "<CAN2_AVM_parking_excute>"
  AVMparkingexcute/1(VHAL_AVMparkingexcute_enum) -> VHAL_AVMparkingexcute_enum/1
  [DT_CAN2_SG_IVI2] -> bus_selector6/1
  bus_selector6/1 -> CAASSw/1(CAAS_Sw)  "<CAN2_CAAS_Sw>"
  CAASSw/1(VHAL_CAASSw_enum) -> VHAL_CAASSw_enum/1
  [DT_CAN2_SG_IVI2] -> bus_selector7/1
  bus_selector7/1 -> CDLLockButt/1(CDL_Lock_Butt)  "<CAN2_CDL_Lock_Butt>"
  CDLLockButt/1(VHAL_CDLLockButt_flg) -> VHAL_CDLLockButt_flg/1
  [DT_CAN2_SG_IVI2] -> bus_selector8/1
  bus_selector8/1 -> CDLUnlockButt/1(CDL_Unlock_Butt)  "<CAN2_CDL_Unlock_Butt>"
  CDLUnlockButt/1(VHAL_CDLUnlockButt_flg) -> VHAL_CDLUnlockButt_flg/1
  [DT_CAN2_SG_IVI2] -> bus_selector9/1
  bus_selector9/1 -> DSEATantiset/1(DSEAT_anti_set)  "<CAN2_DSEAT_anti_set>"
  DSEATantiset/1(VHAL_DSEATantiset_flg) -> VHAL_DSEATantiset_flg/1
  [DT_CAN2_SG_IVI2] -> bus_selector10/1
  bus_selector10/1 -> DSEATentryfunset/1(DSEAT_entryfun_set)  "<CAN2_DSEAT_entryfun_set>"
  DSEATentryfunset/1(VHAL_DSEATentryfunset_flg) -> VHAL_DSEATentryfunset_flg/1
  [DT_CAN2_SG_IVI2] -> bus_selector11/1
  bus_selector11/1 -> DSEATventreq/1(DSEAT_vent_req)  "<CAN2_DSEAT_vent_req>"
  DSEATventreq/1(VHAL_DSEATventreq_enum) -> VHAL_DSEATventreq_enum/1
  [DT_CAN2_SG_IVI2] -> bus_selector12/1
  bus_selector12/1 -> Distanceunit/1(Distance_unit)  "<CAN2_Distance_unit>"
  Distanceunit/1(VHAL_Distanceunit_flg) -> VHAL_Distanceunit_flg/1
  [DT_CAN2_SG_IVI2] -> bus_selector13/1
  bus_selector13/1 -> ESCSWCmd/1(ESC_SW_Cmd)  "<CAN2_ESC_SW_Cmd>"
  ESCSWCmd/1(VHAL_ESCSWCmd_enum) -> VHAL_ESCSWCmd_enum/1
  [DT_CAN2_SG_IVI2] -> bus_selector14/1
  bus_selector14/1 -> FSOffSw/1(FS_Off_Sw)  "<CAN2_FS_Off_Sw>"
  FSOffSw/1(VHAL_FSOffSw_enum) -> VHAL_FSOffSw_enum/1
  [DT_CAN2_SG_IVI2] -> bus_selector15/1
  bus_selector15/1 -> FollowMeSW/1(FollowMeSW)  "<CAN2_FollowMeSW>"
  FollowMeSW/1(VHAL_FollowMeSW_flg) -> VHAL_FollowMeSW_flg/1
  [DT_CAN2_SG_IVI2] -> bus_selector16/1
  bus_selector16/1 -> GPSLAT/1(GPS_LAT)  "<CAN2_GPS_LAT>"
  GPSLAT/1(VHAL_GPSLAT_s) -> VHAL_GPSLAT_s/1
  [DT_CAN2_SG_IVI2] -> bus_selector17/1
  bus_selector17/1 -> GPSLONG/1(GPS_LONG)  "<CAN2_GPS_LONG>"
  GPSLONG/1(VHAL_GPSLONG_enum) -> VHAL_GPSLONG_enum/1
  [DT_CAN2_SG_IVI2] -> bus_selector18/1
  bus_selector18/1 -> HeadLampSW/1(HeadLampSW)  "<CAN2_HeadLampSW>"
  HeadLampSW/1(VHAL_HeadLampSW_enum) -> VHAL_HeadLampSW_enum/1
  [DT_CAN2_SG_IVI2] -> bus_selector19/1
  bus_selector19/1 -> HoodLatchSW/1(Hood_Latch_SW)  "<CAN2_Hood_Latch_SW>"
  HoodLatchSW/1(VHAL_HoodLatchSW_enum) -> VHAL_HoodLatchSW_enum/1
  [DT_CAN2_SG_IVI2] -> bus_selector20/1
  bus_selector20/1 -> IVINightModeSta/1(IVI_Night_Mode_Sta)  "<CAN2_IVI_Night_Mode_Sta>"
  IVINightModeSta/1(VHAL_IVINightModeSta_flg) -> VHAL_IVINightModeSta_flg/1
  [DT_CAN2_SG_IVI2] -> bus_selector21/1
  bus_selector21/1 -> IVIPTGModeSW/1(IVI_PTG_Mode_SW)  "<CAN2_IVI_PTG_Mode_SW>"
  IVIPTGModeSW/1(VHAL_IVIPTGModeSW_enum) -> VHAL_IVIPTGModeSW_enum/1
  [DT_CAN2_SG_IVI2] -> bus_selector22/1
  bus_selector22/1 -> IVIPTGStaSW/1(IVI_PTG_Sta_SW)  "<CAN2_IVI_PTG_Sta_SW>"
  IVIPTGStaSW/1(VHAL_IVIPTGStaSW_enum) -> VHAL_IVIPTGStaSW_enum/1
  [DT_CAN2_SG_IVI2] -> bus_selector23/1
  bus_selector23/1 -> IVIPTGUSStaSW/1(IVI_PTG_USSta_SW)  "<CAN2_IVI_PTG_USSta_SW>"
  IVIPTGUSStaSW/1(VHAL_IVIPTGUSStaSW_flg) -> VHAL_IVIPTGUSStaSW_flg/1
  [DT_CAN2_SG_IVI2] -> bus_selector24/1
  bus_selector24/1 -> IVIPWModeReq/1(IVI_PW_Mode_Req)  "<CAN2_IVI_PW_Mode_Req>"
  IVIPWModeReq/1(VHAL_IVIPWModeReq_enum) -> VHAL_IVIPWModeReq_enum/1
  [DT_CAN2_SG_IVI2] -> bus_selector25/1
  bus_selector25/1 -> IVIPwrLockSW/1(IVI_PwrLockSW)  "<CAN2_IVI_PwrLockSW>"
  IVIPwrLockSW/1(VHAL_IVIPwrLockSW_enum) -> VHAL_IVIPwrLockSW_enum/1
  [DT_CAN2_SG_IVI2] -> bus_selector26/1
  bus_selector26/1 -> IVIPwroffreq/1(IVI_Pwroff_req)  "<CAN2_IVI_Pwroff_req>"
  IVIPwroffreq/1(VHAL_IVIPwroffreq_flg) -> VHAL_IVIPwroffreq_flg/1
  [DT_CAN2_SG_IVI2] -> bus_selector27/1
  bus_selector27/1 -> IVIRRDefReq/1(IVI_RR_Def_Req)  "<CAN2_IVI_RR_Def_Req>"
  IVIRRDefReq/1(VHAL_IVIRRDefReq_flg) -> VHAL_IVIRRDefReq_flg/1
  [DT_CAN2_SG_IVI2] -> bus_selector28/1
  bus_selector28/1 -> IVIReqV2L/1(IVI_Req_V2L)  "<CAN2_IVI_Req_V2L>"
  IVIReqV2L/1(VHAL_IVIReqV2L_enum) -> VHAL_IVIReqV2L_enum/1
  [DT_CAN2_SG_IVI2] -> bus_selector29/1
  bus_selector29/1 -> IVIScreen/1(IVI_Screen)  "<CAN2_IVI_Screen>"
  IVIScreen/1(VHAL_IVIScreen_enum) -> VHAL_IVIScreen_enum/1
  [DT_CAN2_SG_IVI2] -> bus_selector30/1
  bus_selector30/1 -> IVIStartChgreq/1(IVI_Start_Chg_req)  "<CAN2_IVI_Start_Chg_req>"
  IVIStartChgreq/1(VHAL_IVIStartChgreq_flg) -> VHAL_IVIStartChgreq_flg/1
  [DT_CAN2_SG_IVI2] -> bus_selector31/1
  bus_selector31/1 -> IVIStatus/1(IVI_Status)  "<CAN2_IVI_Status>"
  IVIStatus/1(VHAL_IVIStatus_flg) -> VHAL_IVIStatus_flg/1
  [DT_CAN2_SG_IVI2] -> bus_selector32/1
  bus_selector32/1 -> IVIStopChgreq/1(IVI_Stop_Chg_req)  "<CAN2_IVI_Stop_Chg_req>"
  IVIStopChgreq/1(VHAL_IVIStopChgreq_flg) -> VHAL_IVIStopChgreq_flg/1
  [DT_CAN2_SG_IVI2] -> bus_selector33/1
  bus_selector33/1 -> IVITriggerreq/1(IVI_Trigger_req)  "<CAN2_IVI_Trigger_req>"
  IVITriggerreq/1(VHAL_IVITriggerreq_flg) -> VHAL_IVITriggerreq_flg/1
  [DT_CAN2_SG_IVI2] -> bus_selector34/1
  bus_selector34/1 -> IVIUnlockChgreq/1(IVI_Unlock_Chg_req)  "<CAN2_IVI_Unlock_Chg_req>"
  IVIUnlockChgreq/1(VHAL_IVIUnlockChgreq_flg) -> VHAL_IVIUnlockChgreq_flg/1
  [DT_CAN2_SG_IVI2] -> bus_selector35/1
  bus_selector35/1 -> IVIWIMAINSW/1(IVI_WI_MAIN_SW)  "<CAN2_IVI_WI_MAIN_SW>"
  IVIWIMAINSW/1(VHAL_IVIWIMAINSW_flg) -> VHAL_IVIWIMAINSW_flg/1
  [DT_CAN2_SG_IVI2] -> bus_selector36/1
  bus_selector36/1 -> LDrvControlCommand/1(L_Drv_ControlCommand)  "<CAN2_L_Drv_ControlCommand>"
  LDrvControlCommand/1(VHAL_LDrvControlCommand_pct) -> VHAL_LDrvControlCommand_pct/1
  [DT_CAN2_SG_IVI2] -> bus_selector37/1
  bus_selector37/1 -> LPasControlCommand/1(L_Pas_ControlCommand)  "<CAN2_L_Pas_ControlCommand>"
  LPasControlCommand/1(VHAL_LPasControlCommand_pct) -> VHAL_LPasControlCommand_pct/1
  [DT_CAN2_SG_IVI2] -> bus_selector38/1
  bus_selector38/1 -> LRLDControlCommand/1(L_RLD_ControlCommand)  "<CAN2_L_RLD_ControlCommand>"
  LRLDControlCommand/1(VHAL_LRLDControlCommand_pct) -> VHAL_LRLDControlCommand_pct/1
  [DT_CAN2_SG_IVI2] -> bus_selector39/1
  bus_selector39/1 -> LRRDControlCommand/1(L_RRD_ControlCommand)  "<CAN2_L_RRD_ControlCommand>"
  LRRDControlCommand/1(VHAL_LRRDControlCommand_pct) -> VHAL_LRRDControlCommand_pct/1
  [DT_CAN2_SG_IVI2] -> bus_selector40/1
  bus_selector40/1 -> LightShowStartReq/1(Light_ShowStart_Req)  "<CAN2_Light_ShowStart_Req>"
  LightShowStartReq/1(VHAL_LightShowStartReq_flg) -> VHAL_LightShowStartReq_flg/1
  [DT_CAN2_SG_IVI2] -> bus_selector41/1
  bus_selector41/1 -> LightShowStopReq/1(Light_ShowStop_Req)  "<CAN2_Light_ShowStop_Req>"
  LightShowStopReq/1(VHAL_LightShowStopReq_flg) -> VHAL_LightShowStopReq_flg/1
  [DT_CAN2_SG_IVI2] -> bus_selector42/1
  bus_selector42/1 -> MFRDNBrightReq/1(MFRD_N_Bright_Req)  "<CAN2_MFRD_N_Bright_Req>"
  MFRDNBrightReq/1(VHAL_MFRDNBrightReq_pct) -> VHAL_MFRDNBrightReq_pct/1
  [DT_CAN2_SG_IVI2] -> bus_selector43/1
  bus_selector43/1 -> OFFACMODE/1(OFF_AC_MODE)  "<CAN2_OFF_AC_MODE>"
  OFFACMODE/1(VHAL_OFFACMODE_enum) -> VHAL_OFFACMODE_enum/1
  [DT_CAN2_SG_IVI2] -> bus_selector44/1
  bus_selector44/1 -> PSEATventreq/1(PSEAT_vent_req)  "<CAN2_PSEAT_vent_req>"
  PSEATventreq/1(VHAL_PSEATventreq_enum) -> VHAL_PSEATventreq_enum/1
  [DT_CAN2_SG_IVI2] -> bus_selector45/1
  bus_selector45/1 -> PerdV2L/1(Perd_V2L)  "<CAN2_Perd_V2L>"
  PerdV2L/1(VHAL_PerdV2L_enum) -> VHAL_PerdV2L_enum/1
  [DT_CAN2_SG_IVI2] -> bus_selector46/1
  bus_selector46/1 -> RFogLampSW/1(RFogLampSW)  "<CAN2_RFogLampSW>"
  RFogLampSW/1(VHAL_RFogLampSW_flg) -> VHAL_RFogLampSW_flg/1
  [DT_CAN2_SG_IVI2] -> bus_selector47/1
  bus_selector47/1 -> RollModeSWCmd/1(Roll_Mode_SW_Cmd)  "<CAN2_Roll_Mode_SW_Cmd>"
  RollModeSWCmd/1(VHAL_RollModeSWCmd_enum) -> VHAL_RollModeSWCmd_enum/1
  [DT_CAN2_SG_IVI2] -> bus_selector48/1
  bus_selector48/1 -> RoomLampMode/1(RoomLampMode)  "<CAN2_RoomLampMode>"
  RoomLampMode/1(VHAL_RoomLampMode_flg) -> VHAL_RoomLampMode_flg/1
  [DT_CAN2_SG_IVI2] -> bus_selector49/1
  bus_selector49/1 -> SOCADJBUTT/1(SOC_ADJ_BUTT)  "<CAN2_SOC_ADJ_BUTT>"
  SOCADJBUTT/1(VHAL_SOCADJBUTT_flg) -> VHAL_SOCADJBUTT_flg/1
  [DT_CAN2_SG_IVI2] -> bus_selector50/1
  bus_selector50/1 -> SOCLimitSet/1(SOC_Limit_Set)  "<CAN2_SOC_Limit_Set>"
  SOCLimitSet/1(VHAL_SOCLimitSet_pct) -> VHAL_SOCLimitSet_pct/1
  [DT_CAN2_SG_IVI2] -> bus_selector51/1
  bus_selector51/1 -> SOCV2LLimit/1(SOC_V2LLimit)  "<CAN2_SOC_V2LLimit>"
  SOCV2LLimit/1(VHAL_SOCV2LLimit_pct) -> VHAL_SOCV2LLimit_pct/1
  [DT_CAN2_SG_IVI2] -> bus_selector52/1
  bus_selector52/1 -> SchedChgStart/1(Sched_Chg_Start)  "<CAN2_Sched_Chg_Start>"
  SchedChgStart/1(VHAL_SchedChgStart_flg) -> VHAL_SchedChgStart_flg/1
  [DT_CAN2_SG_IVI2] -> bus_selector53/1
  bus_selector53/1 -> SchedChgStop/1(Sched_Chg_Stop)  "<CAN2_Sched_Chg_Stop>"
  SchedChgStop/1(VHAL_SchedChgStop_flg) -> VHAL_SchedChgStop_flg/1
  [DT_CAN2_SG_IVI2] -> bus_selector54/1
  bus_selector54/1 -> SchedChgbutt/1(Sched_Chg_butt)  "<CAN2_Sched_Chg_butt>"
  SchedChgbutt/1(VHAL_SchedChgbutt_flg) -> VHAL_SchedChgbutt_flg/1
  [DT_CAN2_SG_IVI2] -> bus_selector55/1
  bus_selector55/1 -> SchedChglimit/1(Sched_Chg_limit)  "<CAN2_Sched_Chg_limit>"
  SchedChglimit/1(VHAL_SchedChglimit_pct) -> VHAL_SchedChglimit_pct/1
  [DT_CAN2_SG_IVI2] -> bus_selector56/1
  bus_selector56/1 -> SchedChgwake/1(Sched_Chg_wake)  "<CAN2_Sched_Chg_wake>"
  SchedChgwake/1(VHAL_SchedChgwake_flg) -> VHAL_SchedChgwake_flg/1
  [DT_CAN2_SG_IVI2] -> bus_selector57/1
  bus_selector57/1 -> SenstivityPosition/1(SenstivityPosition)  "<CAN2_SenstivityPosition>"
  SenstivityPosition/1(VHAL_SenstivityPosition_enum) -> VHAL_SenstivityPosition_enum/1
  [DT_CAN2_SG_IVI2] -> bus_selector58/1
  bus_selector58/1 -> SetUnlockSingle/1(SetUnlockSingle)  "<CAN2_SetUnlockSingle>"
  SetUnlockSingle/1(VHAL_SetUnlockSingle_flg) -> VHAL_SetUnlockSingle_flg/1
  [DT_CAN2_SG_IVI2] -> bus_selector59/1
  bus_selector59/1 -> TCSSWCmd/1(TCS_SW_Cmd)  "<CAN2_TCS_SW_Cmd>"
  TCSSWCmd/1(VHAL_TCSSWCmd_enum) -> VHAL_TCSSWCmd_enum/1
  [DT_CAN2_SG_IVI2] -> bus_selector60/1
  bus_selector60/1 -> TPMSCaliButt/1(TPMS_Cali_Butt)  "<CAN2_TPMS_Cali_Butt>"
  TPMSCaliButt/1(VHAL_TPMSCaliButt_flg) -> VHAL_TPMSCaliButt_flg/1
  [DT_CAN2_SG_IVI2] -> bus_selector61/1
  bus_selector61/1 -> TPMSResButt/1(TPMS_Res_Butt)  "<CAN2_TPMS_Res_Butt>"
  TPMSResButt/1(VHAL_TPMSResButt_flg) -> VHAL_TPMSResButt_flg/1
  [DT_CAN2_SG_IVI2] -> bus_selector62/1
  bus_selector62/1 -> TurnSwTimeSet/1(TurnSwTimeSet)  "<CAN2_TurnSwTimeSet>"
  TurnSwTimeSet/1(VHAL_TurnSwTimeSet_enum) -> VHAL_TurnSwTimeSet_enum/1
  [DT_CAN2_SG_IVI2] -> bus_selector63/1
  bus_selector63/1 -> WalkawayLockSW/1(Walkaway_Lock_SW)  "<CAN2_Walkaway_Lock_SW>"
  WalkawayLockSW/1(VHAL_WalkawayLockSW_flg) -> VHAL_WalkawayLockSW_flg/1
  [DT_CAN2_SG_IVI2] -> bus_selector64/1
  bus_selector64/1 -> WlcmLightMode/1(WlcmLight_Mode)  "<CAN2_WlcmLight_Mode>"
  WlcmLightMode/1(VHAL_WlcmLightMode_enum) -> VHAL_WlcmLightMode_enum/1
  [DT_CAN2_SG_IVI2] -> bus_selector65/1
  bus_selector65/1 -> sigAirIntenZon1Req/1(sigAirIntenZon1Req)  "<CAN2_sigAirIntenZon1Req>"
  sigAirIntenZon1Req/1(VHAL_sigAirIntenZon1Req_enum) -> VHAL_sigAirIntenZon1Req_enum/1
  [DT_CAN2_SG_IVI2] -> bus_selector66/1
  bus_selector66/1 -> sigDfrstReq/1(sigDfrstReq)  "<CAN2_sigDfrstReq>"
  sigDfrstReq/1(VHAL_sigDfrstReq_flg) -> VHAL_sigDfrstReq_flg/1
  [DT_CAN2_SG_IVI2] -> bus_selector67/1
  bus_selector67/1 -> sigFaceReq/1(sigFaceReq)  "<CAN2_sigFaceReq>"
  sigFaceReq/1(VHAL_sigFaceReq_flg) -> VHAL_sigFaceReq_flg/1
  [DT_CAN2_SG_IVI2] -> bus_selector68/1
  bus_selector68/1 -> sigFootReq/1(sigFootReq)  "<CAN2_sigFootReq>"
  sigFootReq/1(VHAL_sigFootReq_flg) -> VHAL_sigFootReq_flg/1
  [DT_CAN2_SG_IVI2] -> bus_selector69/1
  bus_selector69/1 -> sigRecircReq/1(sigRecircReq)  "<CAN2_sigRecircReq>"
  sigRecircReq/1(VHAL_sigRecircReq_flg) -> VHAL_sigRecircReq_flg/1
  [DT_CAN2_SG_IVI2] -> bus_selector70/1
  bus_selector70/1 -> sigSetTempZon1Req/1(sigSetTempZon1Req)  "<CAN2_sigSetTempZon1Req>"
  sigSetTempZon1Req/1(VHAL_sigSetTempZon1Req_C) -> VHAL_sigSetTempZon1Req_C/1
  [DT_CAN2_SG_IVI2] -> bus_selector71/1
  bus_selector71/1 -> sigSetTempZon2Req/1(sigSetTempZon2Req)  "<CAN2_sigSetTempZon2Req>"
  sigSetTempZon2Req/1(VHAL_sigSetTempZon2Req_C) -> VHAL_sigSetTempZon2Req_C/1

== system halin/HAL_IN/CAN2/IVI_P20_0 ==
  DT_CAN2_SG_IVI_P20_0 : Inport
  IVIFrAtmoLampCmd : Subsystem
  IVIPassengerdoorSta : Subsystem
  IVIRrAtmoLampCmd : Subsystem
  IVIRrRmLampBrightCmd : Subsystem
  IVIRrRoomlampCmd : Subsystem
  bus_selector : BusSelector  OutputSignals=CAN2_IVI_FrAtmoLamp_Cmd
  bus_selector1 : BusSelector  OutputSignals=CAN2_IVI_Passengerdoor_Sta
  bus_selector2 : BusSelector  OutputSignals=CAN2_IVI_RrAtmoLamp_Cmd
  bus_selector3 : BusSelector  OutputSignals=CAN2_IVI_RrRmLampBright_Cmd
  bus_selector4 : BusSelector  OutputSignals=CAN2_IVI_RrRoomlamp_Cmd
  VHAL_IVIFrAtmoLampCmd_flg : Outport
  VHAL_IVIPassengerdoorSta_flg : Outport  Port=2
  VHAL_IVIRrAtmoLampCmd_flg : Outport  Port=3
  VHAL_IVIRrRmLampBrightCmd_enum : Outport  Port=4
  VHAL_IVIRrRoomlampCmd_flg : Outport  Port=5
  wires:
  DT_CAN2_SG_IVI_P20_0/1 -> [DT_CAN2_SG_IVI_P20_0]
  [DT_CAN2_SG_IVI_P20_0] -> bus_selector/1
  bus_selector/1 -> IVIFrAtmoLampCmd/1(IVI_FrAtmoLamp_Cmd)  "<CAN2_IVI_FrAtmoLamp_Cmd>"
  IVIFrAtmoLampCmd/1(VHAL_IVIFrAtmoLampCmd_flg) -> VHAL_IVIFrAtmoLampCmd_flg/1
  [DT_CAN2_SG_IVI_P20_0] -> bus_selector1/1
  bus_selector1/1 -> IVIPassengerdoorSta/1(IVI_Passengerdoor_Sta)  "<CAN2_IVI_Passengerdoor_Sta>"
  IVIPassengerdoorSta/1(VHAL_IVIPassengerdoorSta_flg) -> VHAL_IVIPassengerdoorSta_flg/1
  [DT_CAN2_SG_IVI_P20_0] -> bus_selector2/1
  bus_selector2/1 -> IVIRrAtmoLampCmd/1(IVI_RrAtmoLamp_Cmd)  "<CAN2_IVI_RrAtmoLamp_Cmd>"
  IVIRrAtmoLampCmd/1(VHAL_IVIRrAtmoLampCmd_flg) -> VHAL_IVIRrAtmoLampCmd_flg/1
  [DT_CAN2_SG_IVI_P20_0] -> bus_selector3/1
  bus_selector3/1 -> IVIRrRmLampBrightCmd/1(IVI_RrRmLampBright_Cmd)  "<CAN2_IVI_RrRmLampBright_Cmd>"
  IVIRrRmLampBrightCmd/1(VHAL_IVIRrRmLampBrightCmd_enum) -> VHAL_IVIRrRmLampBrightCmd_enum/1
  [DT_CAN2_SG_IVI_P20_0] -> bus_selector4/1
  bus_selector4/1 -> IVIRrRoomlampCmd/1(IVI_RrRoomlamp_Cmd)  "<CAN2_IVI_RrRoomlamp_Cmd>"
  IVIRrRoomlampCmd/1(VHAL_IVIRrRoomlampCmd_flg) -> VHAL_IVIRrRoomlampCmd_flg/1

== system halin/HAL_IN/CAN2/METER1 ==
  DT_CAN2_SG_METER1 : Inport
  METERKPHCalcu : Subsystem
  ODOMETER : Subsystem
  bus_selector : BusSelector  OutputSignals=CAN2_METER_KPH_Calcu
  bus_selector1 : BusSelector  OutputSignals=CAN2_ODOMETER
  VHAL_METERKPHCalcu_kph : Outport
  VHAL_ODOMETER_km : Outport  Port=2
  wires:
  DT_CAN2_SG_METER1/1 -> [DT_CAN2_SG_METER1]
  [DT_CAN2_SG_METER1] -> bus_selector/1
  bus_selector/1 -> METERKPHCalcu/1(METER_KPH_Calcu)  "<CAN2_METER_KPH_Calcu>"
  METERKPHCalcu/1(VHAL_METERKPHCalcu_kph) -> VHAL_METERKPHCalcu_kph/1
  [DT_CAN2_SG_METER1] -> bus_selector1/1
  bus_selector1/1 -> ODOMETER/1(ODOMETER)  "<CAN2_ODOMETER>"
  ODOMETER/1(VHAL_ODOMETER_km) -> VHAL_ODOMETER_km/1

== system halin/HAL_IN/CAN2/VHAL_CANMsgInvalidIVI1_flg ==
  Cast To Boolean13 : DataTypeConversion  OutDataTypeStr=boolean
  Constant : Constant  Value=TRUE
  Latch13 : hcu_lib/Basic_Blocks/Latch
  Switch13 : Switch  Criteria=u2 ~= 0
  Unit Delay : UnitDelay  SampleTime=-1  HasFrameUpgradeWarning=on
  UnitConverter : DataTypeConversion  OutDataTypeStr=boolean
  Out : Outport
  wires:
  Constant/1 -> Switch13/3
  Unit Delay/1 -> Cast To Boolean13/1
  Cast To Boolean13/1 -> Switch13/1, Latch13/1
  Switch13/1 -> UnitConverter/1
  Latch13/1 -> Switch13/2
  UnitConverter/1 -> Unit Delay/1, Out/1  "VHAL_CANMsgInvalidIVI1_flg"

== system halin/HAL_IN/CAN2/VHAL_CANMsgInvalidIVI2_flg ==
  Cast To Boolean13 : DataTypeConversion  OutDataTypeStr=boolean
  Constant : Constant  Value=TRUE
  Latch13 : hcu_lib/Basic_Blocks/Latch
  Switch13 : Switch  Criteria=u2 ~= 0
  Unit Delay : UnitDelay  SampleTime=-1  HasFrameUpgradeWarning=on
  UnitConverter : DataTypeConversion  OutDataTypeStr=boolean
  Out : Outport
  wires:
  Constant/1 -> Switch13/3
  Unit Delay/1 -> Cast To Boolean13/1
  Cast To Boolean13/1 -> Switch13/1, Latch13/1
  Switch13/1 -> UnitConverter/1
  Latch13/1 -> Switch13/2
  UnitConverter/1 -> Unit Delay/1, Out/1  "VHAL_CANMsgInvalidIVI2_flg"
